simulink model "PubIfDecisionTOS_MDL"  (R2020b)
settings: configuration reference "DspaceConfig" (kept outside this file)
PostLoadFcn:
  | if any(exist('dsrtsu_mdlpostloadfcn', 'file') ~= 0), dsrtsu_mdlpostloadfcn('Execute', bdroot); end
InitFcn:
  | , if any(exist('dsmpb_private', 'file') ~= 0), dsmpb_private('dsmpb_mdlclblib', 'Init', bdroot); end,
undefined symbols (not defined in the file or in its folder): C_TOS_ACCEgoRAxletoFbumplength_m, C_TOS_ACCTargetFront_Flag, C_TOS_AEBJAPedObjDxThre_Val, C_TOS_AEBJAPedObjDyThre_Val, C_TOS_AEBJATargetSize_Val, C_TOS_AEBJAVehObjDxThre_Val, C_TOS_AEBJAVehObjDyThre_Val, C_TOS_AEBJuncPedTargetSize_Val, C_TOS_AEBLatObjDxThre_Val, C_TOS_AEBLatPedDyThre_Val, C_TOS_AEBLatTargetSize_Val, C_TOS_AEBLongTargetInEgoFront_Flag, C_TOS_axAbsGround_Parameter, C_TOS_CameraConfirmedFlag, C_TOS_CNsubjWidth, C_TOS_CurrentLaneCoreMinWidth_Val, C_TOS_CutInProb_Val_Zero, C_TOS_CutOutProb_Val_Zero, C_TOS_D2R_Val, C_TOS_DefaultValueObjectToCenterLine_dy, C_TOS_EgoCarWidth_Val, C_TOS_EgoDxRefPoint_m, C_TOS_EgoRAxletoFbumplength_m, C_TOS_HalfWidthVehicle_Con, C_TOS_HWA_CurrentLaneFlag, C_TOS_HWA_LeftLaneFlag, C_TOS_HWA_MovingDir_Vaild, C_TOS_HWA_MovState_Vaild, C_TOS_HWA_RightLaneFlag, C_TOS_LaneLineCourseErrorFront, C_TOS_LaneLineCourseErrorRear, C_TOS_MotorbikeDefaultWidth_m, C_TOS_NumberOfEffectiveTargets, C_TOS_Obj_Age_Val, C_TOS_Objdx_Constraint_Val, C_TOS_ObjectDefaultWidth_m, C_TOS_ObjInCurrentLane_Val, C_TOS_ObjInCurrentLaneValid, C_TOS_ObjInLeftLaneValid, C_TOS_ObjInRightLaneValid, C_TOS_ObjNotInCurrentLane_Val, C_TOS_ObjNotREElementType, C_TOS_ObjPredictDis_dy_ConstantVal_Zeros, C_TOS_ObjToCenterLine_ConstantVal_Zeros, C_TOS_OFMObjIDInvilad_Val, C_TOS_PIL_LatDisCons_Val_zero, C_TOS_PIL_ObjectCutInFlag_b, C_TOS_PIL_ObjectCutOutFlag_b, C_TOS_PIL_ObjLaneProb_al_Val, C_TOS_PP_ObjFusType_FC_Confirm_b, C_TOS_PP_ObjFusType_FC_FR_Confirm_b, C_TOS_PP_ObjFusType_FR_Confirm_b, C_TOS_RE_80BoolDefault_Val, C_TOS_RE_80Single181Default_Val, C_TOS_RE_80Single255Default_Val, C_TOS_RE_80Uint8Default_Val, C_TOS_RE_D2R, C_TOS_RE_D_180_Val, C_TOS_RE_InvalidObjectID_Val, C_TOS_RE_InvalidTargetChainDir_Val ... (+142)
libraries: simulink x1650, TOS_LIB x361, canfdmsglib x14
(part 32 of 69)

== system PubIfDecisionTOS_MDL/TOS_20201112/TOS_2012080320/PIL_1029/BoundaryCalculat/ObjectToCenterLine_dyc/RightLane/RightCenterLine_dyc/ObjToCenterLine_dyc_RightLane/line01_dy ==
  Object_DX : Inport
  line01_C0 : Inport  Port=2
  line01_C1 : Inport  Port=3
  line01_C2 : Inport  Port=4
  line01_C3 : Inport  Port=5
  Add : Sum
  Add1 : Sum
  Add3 : Sum
  Constant1 : Constant  Value=3  OutDataTypeStr=single
  Math Function1 : Math  Operator=pow  SignedPower=on  SaturateOnIntegerOverflow=on
  Product : Product
  Product1 : Product
  Product2 : Product
  Square : Math  Operator=square  SignedPower=on  SaturateOnIntegerOverflow=on
  line01_dy : Outport
  wires:
  line01_C1/1 -> Product1/2
  line01_C3/1 -> Product2/2
  Add3/1 -> line01_dy/1
  Add/1 -> Add3/1
  Constant1/1 -> Math Function1/2
  Product1/1 -> Add1/2
  Product2/1 -> Add3/2
  Math Function1/1 -> Product2/1
  Object_DX/1 -> Math Function1/1, Square/1, Product1/1
  Square/1 -> Product/1
  line01_C2/1 -> Product/2
  Product/1 -> Add/2
  line01_C0/1 -> Add1/1
  Add1/1 -> Add/1

== system PubIfDecisionTOS_MDL/TOS_20201112/TOS_2012080320/PIL_1029/BoundaryCalculat/ObjectToCenterLine_dyc/RightLane/RightCenterLine_dyc/ObjToCenterLine_dyc_RightLane/line02_DisJudge ==
  Object_DX : Inport
  line02_dDisStart : Inport  Port=2
  line02_dDisEnd : Inport  Port=3
  Logical Operator : Logic  AllPortsSameDT=off  OutDataTypeStr=boolean
  Relational Operator : RelationalOperator  OutDataTypeStr=boolean  RndMeth=Nearest
  Relational Operator1 : RelationalOperator  Operator=<  OutDataTypeStr=boolean  RndMeth=Nearest
  line02_DisJudge : Outport
  wires:
  Logical Operator/1 -> line02_DisJudge/1
  Relational Operator1/1 -> Logical Operator/2
  Relational Operator/1 -> Logical Operator/1
  Object_DX/1 -> Relational Operator/1, Relational Operator1/1
  line02_dDisStart/1 -> Relational Operator/2
  line02_dDisEnd/1 -> Relational Operator1/2

== system PubIfDecisionTOS_MDL/TOS_20201112/TOS_2012080320/PIL_1029/BoundaryCalculat/ObjectToCenterLine_dyc/RightLane/RightCenterLine_dyc/ObjToCenterLine_dyc_RightLane/line02_dy ==
  Object_DX : Inport
  line02_C0 : Inport  Port=2
  line02_C1 : Inport  Port=3
  line02_C2 : Inport  Port=4
  line02_C3 : Inport  Port=5
  Add : Sum
  Add1 : Sum
  Add3 : Sum
  Constant1 : Constant  Value=3  OutDataTypeStr=single
  Math Function1 : Math  Operator=pow  SignedPower=on  SaturateOnIntegerOverflow=on
  Product : Product
  Product1 : Product
  Product2 : Product
  Square : Math  Operator=square  SignedPower=on  SaturateOnIntegerOverflow=on
  line02_dy : Outport
  wires:
  Add1/1 -> Add/1
  line02_C0/1 -> Add1/1
  Product/1 -> Add/2
  line02_C2/1 -> Product/2
  Square/1 -> Product/1
  Object_DX/1 -> Product1/1, Square/1, Math Function1/1
  Math Function1/1 -> Product2/1
  Product2/1 -> Add3/2
  Product1/1 -> Add1/2
  Constant1/1 -> Math Function1/2
  Add/1 -> Add3/1
  Add3/1 -> line02_dy/1
  line02_C3/1 -> Product2/2
  line02_C1/1 -> Product1/2

== system PubIfDecisionTOS_MDL/TOS_20201112/TOS_2012080320/PIL_1029/BoundaryCalculat/ObjectToCenterLine_dyc/RightLane/RightCenterLine_dyc/ObjToCenterLine_dyc_RightLane/line03_DisJudge ==
  Object_DX : Inport
  line03_dDisStart : Inport  Port=2
  line03_dDisEnd : Inport  Port=3
  Logical Operator : Logic  AllPortsSameDT=off  OutDataTypeStr=boolean
  Relational Operator : RelationalOperator  OutDataTypeStr=boolean  RndMeth=Nearest
  Relational Operator1 : RelationalOperator  Operator=<  OutDataTypeStr=boolean  RndMeth=Nearest
  line03_DisJudge : Outport
  wires:
  line03_dDisEnd/1 -> Relational Operator1/2
  line03_dDisStart/1 -> Relational Operator/2
  Object_DX/1 -> Relational Operator1/1, Relational Operator/1
  Relational Operator/1 -> Logical Operator/1
  Relational Operator1/1 -> Logical Operator/2
  Logical Operator/1 -> line03_DisJudge/1

== system PubIfDecisionTOS_MDL/TOS_20201112/TOS_2012080320/PIL_1029/BoundaryCalculat/ObjectToCenterLine_dyc/RightLane/RightCenterLine_dyc/ObjToCenterLine_dyc_RightLane/line03_dy ==
  Object_DX : Inport
  line03_C0 : Inport  Port=2
  line03_C1 : Inport  Port=3
  line03_C2 : Inport  Port=4
  line03_C3 : Inport  Port=5
  Add : Sum
  Add1 : Sum
  Add3 : Sum
  Constant1 : Constant  Value=3  OutDataTypeStr=single
  Math Function1 : Math  Operator=pow  SignedPower=on  SaturateOnIntegerOverflow=on
  Product : Product
  Product1 : Product
  Product2 : Product
  Square : Math  Operator=square  SignedPower=on  SaturateOnIntegerOverflow=on
  line03_dy : Outport
  wires:
  line03_C1/1 -> Product1/2
  line03_C3/1 -> Product2/2
  Add3/1 -> line03_dy/1
  Add/1 -> Add3/1
  Constant1/1 -> Math Function1/2
  Product1/1 -> Add1/2
  Product2/1 -> Add3/2
  Math Function1/1 -> Product2/1
  Object_DX/1 -> Math Function1/1, Square/1, Product1/1
  Square/1 -> Product/1
  line03_C2/1 -> Product/2
  Product/1 -> Add/2
  line03_C0/1 -> Add1/1
  Add1/1 -> Add/1

== system PubIfDecisionTOS_MDL/TOS_20201112/TOS_2012080320/PIL_1029/BoundaryCalculat/ObjectToCenterLine_dyc/RightLane/RightCenterLine_dyc/ObjToCenterLine_dyc_RightLane/line04_DisJudge ==
  Object_DX : Inport
  line04_dDisStart : Inport  Port=2
  line04_dDisEnd : Inport  Port=3
  Logical Operator : Logic  AllPortsSameDT=off  OutDataTypeStr=boolean
  Relational Operator : RelationalOperator  OutDataTypeStr=boolean  RndMeth=Nearest
  Relational Operator1 : RelationalOperator  Operator=<  OutDataTypeStr=boolean  RndMeth=Nearest
  line04_DisJudge : Outport
  wires:
  Logical Operator/1 -> line04_DisJudge/1
  Relational Operator1/1 -> Logical Operator/2
  Relational Operator/1 -> Logical Operator/1
  Object_DX/1 -> Relational Operator/1, Relational Operator1/1
  line04_dDisStart/1 -> Relational Operator/2
  line04_dDisEnd/1 -> Relational Operator1/2

== system PubIfDecisionTOS_MDL/TOS_20201112/TOS_2012080320/PIL_1029/BoundaryCalculat/ObjectToCenterLine_dyc/RightLane/RightCenterLine_dyc/ObjToCenterLine_dyc_RightLane/line04_dy ==
  Object_DX : Inport
  line04_C0 : Inport  Port=2
  line04_C1 : Inport  Port=3
  line04_C2 : Inport  Port=4
  line04_C3 : Inport  Port=5
  Add : Sum
  Add1 : Sum
  Add3 : Sum
  Constant1 : Constant  Value=3  OutDataTypeStr=single
  Math Function1 : Math  Operator=pow  SignedPower=on  SaturateOnIntegerOverflow=on
  Product : Product
  Product1 : Product
  Product2 : Product
  Square : Math  Operator=square  SignedPower=on  SaturateOnIntegerOverflow=on
  line04_dy : Outport
  wires:
  Add1/1 -> Add/1
  line04_C0/1 -> Add1/1
  Product/1 -> Add/2
  line04_C2/1 -> Product/2
  Square/1 -> Product/1
  Object_DX/1 -> Product1/1, Square/1, Math Function1/1
  Math Function1/1 -> Product2/1
  Product2/1 -> Add3/2
  Product1/1 -> Add1/2
  Constant1/1 -> Math Function1/2
  Add/1 -> Add3/1
  Add3/1 -> line04_dy/1
  line04_C3/1 -> Product2/2
  line04_C1/1 -> Product1/2

== system PubIfDecisionTOS_MDL/TOS_20201112/TOS_2012080320/PIL_1029/BoundaryCalculat/ObjectToCenterLine_dyc/RightLane/RightCenterLine_dyc/ObjToCenterLine_dyc_RightLane/line05_DisJudge ==
  Object_DX : Inport
  line05_dDisStart : Inport  Port=2
  line05_dDisEnd : Inport  Port=3
  Logical Operator : Logic  AllPortsSameDT=off  OutDataTypeStr=boolean
  Relational Operator : RelationalOperator  OutDataTypeStr=boolean  RndMeth=Nearest
  Relational Operator1 : RelationalOperator  Operator=<  OutDataTypeStr=boolean  RndMeth=Nearest
  line05_DisJudge : Outport
  wires:
  line05_dDisEnd/1 -> Relational Operator1/2
  line05_dDisStart/1 -> Relational Operator/2
  Object_DX/1 -> Relational Operator1/1, Relational Operator/1
  Relational Operator/1 -> Logical Operator/1
  Relational Operator1/1 -> Logical Operator/2
  Logical Operator/1 -> line05_DisJudge/1

== system PubIfDecisionTOS_MDL/TOS_20201112/TOS_2012080320/PIL_1029/BoundaryCalculat/ObjectToCenterLine_dyc/RightLane/RightCenterLine_dyc/ObjToCenterLine_dyc_RightLane/line05_dy ==
  Object_DX : Inport
  line05_C0 : Inport  Port=2
  line05_C1 : Inport  Port=3
  line05_C2 : Inport  Port=4
  line05_C3 : Inport  Port=5
  Add : Sum
  Add1 : Sum
  Add3 : Sum
  Constant1 : Constant  Value=3  OutDataTypeStr=single
  Math Function1 : Math  Operator=pow  SignedPower=on  SaturateOnIntegerOverflow=on
  Product : Product
  Product1 : Product
  Product2 : Product
  Square : Math  Operator=square  SignedPower=on  SaturateOnIntegerOverflow=on
  line05_dy : Outport
  wires:
  line05_C1/1 -> Product1/2
  line05_C3/1 -> Product2/2
  Add3/1 -> line05_dy/1
  Add/1 -> Add3/1
  Constant1/1 -> Math Function1/2
  Product1/1 -> Add1/2
  Product2/1 -> Add3/2
  Math Function1/1 -> Product2/1
  Object_DX/1 -> Math Function1/1, Square/1, Product1/1
  Square/1 -> Product/1
  line05_C2/1 -> Product/2
  Product/1 -> Add/2
  line05_C0/1 -> Add1/1
  Add1/1 -> Add/1

== system PubIfDecisionTOS_MDL/TOS_20201112/TOS_2012080320/PIL_1029/BoundaryCalculat/ObjectToCenterLine_dyc/RightLane/RightCenterLine_dyc/ObjToCenterLine_dyc_RightLane/line06_DisJudge ==
  Object_DX : Inport
  line06_dDisStart : Inport  Port=2
  line06_dDisEnd : Inport  Port=3
  Logical Operator : Logic  AllPortsSameDT=off  OutDataTypeStr=boolean
  Relational Operator : RelationalOperator  OutDataTypeStr=boolean  RndMeth=Nearest
  Relational Operator1 : RelationalOperator  Operator=<  OutDataTypeStr=boolean  RndMeth=Nearest
  line06_DisJudge : Outport
  wires:
  Logical Operator/1 -> line06_DisJudge/1
  Relational Operator1/1 -> Logical Operator/2
  Relational Operator/1 -> Logical Operator/1
  Object_DX/1 -> Relational Operator/1, Relational Operator1/1
  line06_dDisStart/1 -> Relational Operator/2
  line06_dDisEnd/1 -> Relational Operator1/2

== system PubIfDecisionTOS_MDL/TOS_20201112/TOS_2012080320/PIL_1029/BoundaryCalculat/ObjectToCenterLine_dyc/RightLane/RightCenterLine_dyc/ObjToCenterLine_dyc_RightLane/line06_dy ==
  Object_DX : Inport
  line06_C0 : Inport  Port=2
  line06_C1 : Inport  Port=3
  line06_C2 : Inport  Port=4
  line6_C3 : Inport  Port=5
  Add : Sum
  Add1 : Sum
  Add3 : Sum
  Constant1 : Constant  Value=3  OutDataTypeStr=single
  Math Function1 : Math  Operator=pow  SignedPower=on  SaturateOnIntegerOverflow=on
  Product : Product
  Product1 : Product
  Product2 : Product
  Square : Math  Operator=square  SignedPower=on  SaturateOnIntegerOverflow=on
  line6_dy : Outport
  wires:
  Add1/1 -> Add/1
  line06_C0/1 -> Add1/1
  Product/1 -> Add/2
  line06_C2/1 -> Product/2
  Square/1 -> Product/1
  Object_DX/1 -> Product1/1, Square/1, Math Function1/1
  Math Function1/1 -> Product2/1
  Product2/1 -> Add3/2
  Product1/1 -> Add1/2
  Constant1/1 -> Math Function1/2
  Add/1 -> Add3/1
  Add3/1 -> line6_dy/1
  line6_C3/1 -> Product2/2
  line06_C1/1 -> Product1/2

== system PubIfDecisionTOS_MDL/TOS_20201112/TOS_2012080320/PIL_1029/BoundaryCalculat/ObjectToCenterLine_dyc/SameLane/PIL_ObjectToCenterLine_dy_Filt/PIL_ObjectToCenterLine_dy/PP_SignalProcessingDefault ==
  Action Port : ActionPort  ActionPortLabel=if(u1 ~= 0)
  Constant : Constant  Value=0  OutDataTypeStr=uint8
  Constant1 : Constant  Value=255  OutDataTypeStr=single
  Obj_ID : Outport
  ObjectToCenterLine_dy_Filt : Outport  Port=2  OutDataTypeStr=single
  wires:
  Constant1/1 -> ObjectToCenterLine_dy_Filt/1
  Constant/1 -> Obj_ID/1

== system PubIfDecisionTOS_MDL/TOS_20201112/TOS_2012080320/PIL_1029/BoundaryCalculat/ObjectToCenterLine_dyc/SameLane/PIL_ObjectToCenterLine_dy_Filt/PIL_ObjectToCenterLine_dy/Subsystem ==
  ObjectID_Filt_K1 : Inport
  ObjectToCenterLine_dy_Filt_K1 : Inport  Port=2  OutDataTypeStr=single
  ObjectToCenterLine_dy : Inport  Port=3  OutDataTypeStr=single
  Object_ID : Inport  Port=4  OutDataTypeStr=uint8
  Object_Age : Inport  Port=5
  TOS_OFMObjValid_Flag : Inport  Port=6
  Action Port : ActionPort  ActionPortLabel=else
  Constant1 : Constant  Value=C_TOS_NumberOfEffectiveTargets  OutDataTypeStr=int32
      settings: AttributesFormatString=C_TOS_NumberOfEffectiveTargets = 80
  Constant2 : Constant  Value=0.2  OutDataTypeStr=single
      settings: AttributesFormatString=P_TOS_PIL_ObjectToCenterLine_dy_CutInDeclineLimit = 0.1
  Constant8 : Constant  Value=0.35  OutDataTypeStr=single
      settings: AttributesFormatString=P_TOS_PIL_ObjectToCenterLine_dy_CutInUpperLimit = 0.5
  ObjectToCenterLine_dyFilit : MATLAB Function  TreatAsAtomicUnit=on
  Terminator : Terminator
  Obj_ID : Outport
  ObjectToCenterLine_dy_Filt : Outport  Port=2  OutDataTypeStr=single
  wires:
  TOS_OFMObjValid_Flag/1 -> ObjectToCenterLine_dyFilit/5(TOS_OFMObjValid_Flag)
  Object_Age/1 -> Terminator/1
  ObjectToCenterLine_dy_Filt_K1/1 -> ObjectToCenterLine_dyFilit/2(ObjectToCenterLine_dy_Filt_K1)
  Object_ID/1 -> Obj_ID/1, ObjectToCenterLine_dyFilit/4(Object_ID)
  ObjectID_Filt_K1/1 -> ObjectToCenterLine_dyFilit/1(ObjectID_Filt_K1)
  Constant2/1 -> ObjectToCenterLine_dyFilit/7(P_TOS_PIL_ObjectToCenterLine_dy_CutInDeclineLimit)
  Constant1/1 -> ObjectToCenterLine_dyFilit/8(Iterator_Num)
  ObjectToCenterLine_dy/1 -> ObjectToCenterLine_dyFilit/3(ObjectToCenterLine_dy)
  Constant8/1 -> ObjectToCenterLine_dyFilit/6(P_TOS_PIL_ObjectToCenterLine_dy_CutInUpperLimit)
  ObjectToCenterLine_dyFilit/1(ObjectToCenterLine_dy_Filt) -> ObjectToCenterLine_dy_Filt/1

== system PubIfDecisionTOS_MDL/TOS_20201112/TOS_2012080320/PIL_1029/BoundaryCalculat/ObjectToCenterLine_dyc/SameLane/SameCenterLine_dyc/ObjToCenterLine_dyc_CurrentLane/line01_DisJudge ==
  Object_DX : Inport
  line01_dDisStart : Inport  Port=2
  line01_dDisEnd : Inport  Port=3
  Logical Operator : Logic  AllPortsSameDT=off  OutDataTypeStr=boolean
  Relational Operator : RelationalOperator  OutDataTypeStr=boolean  RndMeth=Nearest
  Relational Operator1 : RelationalOperator  Operator=<  OutDataTypeStr=boolean  RndMeth=Nearest
  line01_DisJudge : Outport
  wires:
  Logical Operator/1 -> line01_DisJudge/1
  Relational Operator1/1 -> Logical Operator/2
  Relational Operator/1 -> Logical Operator/1
  Object_DX/1 -> Relational Operator/1, Relational Operator1/1
  line01_dDisStart/1 -> Relational Operator/2
  line01_dDisEnd/1 -> Relational Operator1/2

== system PubIfDecisionTOS_MDL/TOS_20201112/TOS_2012080320/PIL_1029/BoundaryCalculat/ObjectToCenterLine_dyc/SameLane/SameCenterLine_dyc/ObjToCenterLine_dyc_CurrentLane/line01_dy ==
  Object_DX : Inport
  line01_C0 : Inport  Port=2
  line01_C1 : Inport  Port=3
  line01_C2 : Inport  Port=4
  line01_C3 : Inport  Port=5
  Add : Sum
  Add1 : Sum
  Add3 : Sum
  Constant1 : Constant  Value=3  OutDataTypeStr=single
  Math Function1 : Math  Operator=pow  SignedPower=on  SaturateOnIntegerOverflow=on
  Product : Product
  Product1 : Product
  Product2 : Product
  Square : Math  Operator=square  SignedPower=on  SaturateOnIntegerOverflow=on
  line01_dy : Outport
  wires:
  Add1/1 -> Add/1
  line01_C0/1 -> Add1/1
  Product/1 -> Add/2
  line01_C2/1 -> Product/2
  Square/1 -> Product/1
  Object_DX/1 -> Product1/1, Square/1, Math Function1/1
  Math Function1/1 -> Product2/1
  Product2/1 -> Add3/2
  Product1/1 -> Add1/2
  Constant1/1 -> Math Function1/2
  Add/1 -> Add3/1
  Add3/1 -> line01_dy/1
  line01_C3/1 -> Product2/2
  line01_C1/1 -> Product1/2

== system PubIfDecisionTOS_MDL/TOS_20201112/TOS_2012080320/PIL_1029/BoundaryCalculat/ObjectToCenterLine_dyc/SameLane/SameCenterLine_dyc/ObjToCenterLine_dyc_CurrentLane/line02_DisJudge ==
  Object_DX : Inport
  line02_dDisStart : Inport  Port=2
  line02_dDisEnd : Inport  Port=3
  Logical Operator : Logic  AllPortsSameDT=off  OutDataTypeStr=boolean
  Relational Operator : RelationalOperator  OutDataTypeStr=boolean  RndMeth=Nearest
  Relational Operator1 : RelationalOperator  Operator=<  OutDataTypeStr=boolean  RndMeth=Nearest
  line02_DisJudge : Outport
  wires:
  line02_dDisEnd/1 -> Relational Operator1/2
  line02_dDisStart/1 -> Relational Operator/2
  Object_DX/1 -> Relational Operator1/1, Relational Operator/1
  Relational Operator/1 -> Logical Operator/1
  Relational Operator1/1 -> Logical Operator/2
  Logical Operator/1 -> line02_DisJudge/1

== system PubIfDecisionTOS_MDL/TOS_20201112/TOS_2012080320/PIL_1029/BoundaryCalculat/ObjectToCenterLine_dyc/SameLane/SameCenterLine_dyc/ObjToCenterLine_dyc_CurrentLane/line02_dy ==
  Object_DX : Inport
  line02_C0 : Inport  Port=2
  line02_C1 : Inport  Port=3
  line02_C2 : Inport  Port=4
  line02_C3 : Inport  Port=5
  Add : Sum
  Add1 : Sum
  Add3 : Sum
  Constant1 : Constant  Value=3  OutDataTypeStr=single
  Math Function1 : Math  Operator=pow  SignedPower=on  SaturateOnIntegerOverflow=on
  Product : Product
  Product1 : Product
  Product2 : Product
  Square : Math  Operator=square  SignedPower=on  SaturateOnIntegerOverflow=on
  line02_dy : Outport
  wires:
  line02_C1/1 -> Product1/2
  line02_C3/1 -> Product2/2
  Add3/1 -> line02_dy/1
  Add/1 -> Add3/1
  Constant1/1 -> Math Function1/2
  Product1/1 -> Add1/2
  Product2/1 -> Add3/2
  Math Function1/1 -> Product2/1
  Object_DX/1 -> Math Function1/1, Square/1, Product1/1
  Square/1 -> Product/1
  line02_C2/1 -> Product/2
  Product/1 -> Add/2
  line02_C0/1 -> Add1/1
  Add1/1 -> Add/1

== system PubIfDecisionTOS_MDL/TOS_20201112/TOS_2012080320/PIL_1029/BoundaryCalculat/ObjectToCenterLine_dyc/SameLane/SameCenterLine_dyc/ObjToCenterLine_dyc_CurrentLane/line03_DisJudge ==
  Object_DX : Inport
  line03_dDisStart : Inport  Port=2
  line03_dDisEnd : Inport  Port=3
  Logical Operator : Logic  AllPortsSameDT=off  OutDataTypeStr=boolean
  Relational Operator : RelationalOperator  OutDataTypeStr=boolean  RndMeth=Nearest
  Relational Operator1 : RelationalOperator  Operator=<  OutDataTypeStr=boolean  RndMeth=Nearest
  line03_DisJudge : Outport
  wires:
  Logical Operator/1 -> line03_DisJudge/1
  Relational Operator1/1 -> Logical Operator/2
  Relational Operator/1 -> Logical Operator/1
  Object_DX/1 -> Relational Operator/1, Relational Operator1/1
  line03_dDisStart/1 -> Relational Operator/2
  line03_dDisEnd/1 -> Relational Operator1/2

== system PubIfDecisionTOS_MDL/TOS_20201112/TOS_2012080320/PIL_1029/BoundaryCalculat/ObjectToCenterLine_dyc/SameLane/SameCenterLine_dyc/ObjToCenterLine_dyc_CurrentLane/line03_dy ==
  Object_DX : Inport
  line03_C0 : Inport  Port=2
  line03_C1 : Inport  Port=3
  line03_C2 : Inport  Port=4
  line03_C3 : Inport  Port=5
  Add : Sum
  Add1 : Sum
  Add3 : Sum
  Constant1 : Constant  Value=3  OutDataTypeStr=single
  Math Function1 : Math  Operator=pow  SignedPower=on  SaturateOnIntegerOverflow=on
  Product : Product
  Product1 : Product
  Product2 : Product
  Square : Math  Operator=square  SignedPower=on  SaturateOnIntegerOverflow=on
  line03_dy : Outport
  wires:
  Add1/1 -> Add/1
  line03_C0/1 -> Add1/1
  Product/1 -> Add/2
  line03_C2/1 -> Product/2
  Square/1 -> Product/1
  Object_DX/1 -> Product1/1, Square/1, Math Function1/1
  Math Function1/1 -> Product2/1
  Product2/1 -> Add3/2
  Product1/1 -> Add1/2
  Constant1/1 -> Math Function1/2
  Add/1 -> Add3/1
  Add3/1 -> line03_dy/1
  line03_C3/1 -> Product2/2
  line03_C1/1 -> Product1/2

== system PubIfDecisionTOS_MDL/TOS_20201112/TOS_2012080320/PIL_1029/BoundaryCalculat/ObjectToCenterLine_dyc/SameLane/SameCenterLine_dyc/ObjToCenterLine_dyc_CurrentLane/line04_DisJudge ==
  Object_DX : Inport
  line04_dDisStart : Inport  Port=2
  line04_dDisEnd : Inport  Port=3
  Logical Operator : Logic  AllPortsSameDT=off  OutDataTypeStr=boolean
  Relational Operator : RelationalOperator  OutDataTypeStr=boolean  RndMeth=Nearest
  Relational Operator1 : RelationalOperator  Operator=<  OutDataTypeStr=boolean  RndMeth=Nearest
  line04_DisJudge : Outport
  wires:
  line04_dDisEnd/1 -> Relational Operator1/2
  line04_dDisStart/1 -> Relational Operator/2
  Object_DX/1 -> Relational Operator1/1, Relational Operator/1
  Relational Operator/1 -> Logical Operator/1
  Relational Operator1/1 -> Logical Operator/2
  Logical Operator/1 -> line04_DisJudge/1

== system PubIfDecisionTOS_MDL/TOS_20201112/TOS_2012080320/PIL_1029/BoundaryCalculat/ObjectToCenterLine_dyc/SameLane/SameCenterLine_dyc/ObjToCenterLine_dyc_CurrentLane/line04_dy ==
  Object_DX : Inport
  line04_C0 : Inport  Port=2
  line04_C1 : Inport  Port=3
  line04_C2 : Inport  Port=4
  line04_C3 : Inport  Port=5
  Add : Sum
  Add1 : Sum
  Add3 : Sum
  Constant1 : Constant  Value=3  OutDataTypeStr=single
  Math Function1 : Math  Operator=pow  SignedPower=on  SaturateOnIntegerOverflow=on
  Product : Product
  Product1 : Product
  Product2 : Product
  Square : Math  Operator=square  SignedPower=on  SaturateOnIntegerOverflow=on
  line04_dy : Outport
  wires:
  line04_C1/1 -> Product1/2
  line04_C3/1 -> Product2/2
  Add3/1 -> line04_dy/1
  Add/1 -> Add3/1
  Constant1/1 -> Math Function1/2
  Product1/1 -> Add1/2
  Product2/1 -> Add3/2
  Math Function1/1 -> Product2/1
  Object_DX/1 -> Math Function1/1, Square/1, Product1/1
  Square/1 -> Product/1
  line04_C2/1 -> Product/2
  Product/1 -> Add/2
  line04_C0/1 -> Add1/1
  Add1/1 -> Add/1

== system PubIfDecisionTOS_MDL/TOS_20201112/TOS_2012080320/PIL_1029/BoundaryCalculat/ObjectToCenterLine_dyc/SameLane/SameCenterLine_dyc/ObjToCenterLine_dyc_CurrentLane/line05_DisJudge ==
  Object_DX : Inport
  line05_dDisStart : Inport  Port=2
  line05_dDisEnd : Inport  Port=3
  Logical Operator : Logic  AllPortsSameDT=off  OutDataTypeStr=boolean
  Relational Operator : RelationalOperator  OutDataTypeStr=boolean  RndMeth=Nearest
  Relational Operator1 : RelationalOperator  Operator=<  OutDataTypeStr=boolean  RndMeth=Nearest
  line05_DisJudge : Outport
  wires:
  Logical Operator/1 -> line05_DisJudge/1
  Relational Operator1/1 -> Logical Operator/2
  Relational Operator/1 -> Logical Operator/1
  Object_DX/1 -> Relational Operator/1, Relational Operator1/1
  line05_dDisStart/1 -> Relational Operator/2
  line05_dDisEnd/1 -> Relational Operator1/2

== system PubIfDecisionTOS_MDL/TOS_20201112/TOS_2012080320/PIL_1029/BoundaryCalculat/ObjectToCenterLine_dyc/SameLane/SameCenterLine_dyc/ObjToCenterLine_dyc_CurrentLane/line05_dy ==
  Object_DX : Inport
  line05_C0 : Inport  Port=2
  line05_C1 : Inport  Port=3
  line05_C2 : Inport  Port=4
  line05_C3 : Inport  Port=5
  Add : Sum
  Add1 : Sum
  Add3 : Sum
  Constant1 : Constant  Value=3  OutDataTypeStr=single
  Math Function1 : Math  Operator=pow  SignedPower=on  SaturateOnIntegerOverflow=on
  Product : Product
  Product1 : Product
  Product2 : Product
  Square : Math  Operator=square  SignedPower=on  SaturateOnIntegerOverflow=on
  line05_dy : Outport
  wires:
  Add1/1 -> Add/1
  line05_C0/1 -> Add1/1
  Product/1 -> Add/2
  line05_C2/1 -> Product/2
  Square/1 -> Product/1
  Object_DX/1 -> Product1/1, Square/1, Math Function1/1
  Math Function1/1 -> Product2/1
  Product2/1 -> Add3/2
  Product1/1 -> Add1/2
  Constant1/1 -> Math Function1/2
  Add/1 -> Add3/1
  Add3/1 -> line05_dy/1
  line05_C3/1 -> Product2/2
  line05_C1/1 -> Product1/2

== system PubIfDecisionTOS_MDL/TOS_20201112/TOS_2012080320/PIL_1029/BoundaryCalculat/ObjectToCenterLine_dyc/SameLane/SameCenterLine_dyc/ObjToCenterLine_dyc_CurrentLane/line06_DisJudge ==
  Object_DX : Inport
  line06_dDisStart : Inport  Port=2
  line06_dDisEnd : Inport  Port=3
  Logical Operator : Logic  AllPortsSameDT=off  OutDataTypeStr=boolean
  Relational Operator : RelationalOperator  OutDataTypeStr=boolean  RndMeth=Nearest
  Relational Operator1 : RelationalOperator  Operator=<  OutDataTypeStr=boolean  RndMeth=Nearest
  line06_DisJudge : Outport
  wires:
  line06_dDisEnd/1 -> Relational Operator1/2
  line06_dDisStart/1 -> Relational Operator/2
  Object_DX/1 -> Relational Operator1/1, Relational Operator/1
  Relational Operator/1 -> Logical Operator/1
  Relational Operator1/1 -> Logical Operator/2
  Logical Operator/1 -> line06_DisJudge/1

== system PubIfDecisionTOS_MDL/TOS_20201112/TOS_2012080320/PIL_1029/BoundaryCalculat/ObjectToCenterLine_dyc/SameLane/SameCenterLine_dyc/ObjToCenterLine_dyc_CurrentLane/line06_dy ==
  Object_DX : Inport
  line06_C0 : Inport  Port=2
  line06_C1 : Inport  Port=3
  line06_C2 : Inport  Port=4
  line6_C3 : Inport  Port=5
  Add : Sum
  Add1 : Sum
  Add3 : Sum
  Constant1 : Constant  Value=3  OutDataTypeStr=single
  Math Function1 : Math  Operator=pow  SignedPower=on  SaturateOnIntegerOverflow=on
  Product : Product
  Product1 : Product
  Product2 : Product
  Square : Math  Operator=square  SignedPower=on  SaturateOnIntegerOverflow=on
  line6_dy : Outport
  wires:
  line06_C1/1 -> Product1/2
  line6_C3/1 -> Product2/2
  Add3/1 -> line6_dy/1
  Add/1 -> Add3/1
  Constant1/1 -> Math Function1/2
  Product1/1 -> Add1/2
  Product2/1 -> Add3/2
  Math Function1/1 -> Product2/1
  Object_DX/1 -> Math Function1/1, Square/1, Product1/1
  Square/1 -> Product/1
  line06_C2/1 -> Product/2
  Product/1 -> Add/2
  line06_C0/1 -> Add1/1
  Add1/1 -> Add/1

== system PubIfDecisionTOS_MDL/TOS_20201112/TOS_2012080320/PIL_1029/ObjCutInOut_Prob/ObjectCutIn/CutInProb_Calculate/CutInProb_Calculate_/CutInPredictDis_dy/CutInPredictTime ==
  note: 非车辆目标，根据 ObjectToCenterLine_dy 定义预测时间
  ObjectToCenterLine_dy_Filt : Inport  OutDataTypeStr=single
  ObjectToCenterLine_dy : Inport  Port=2  OutDataTypeStr=single
  ObjectType : Inport  Port=3
  PP_ObjectToCenterLine_vyc : Inport  Port=4  OutDataTypeStr=single
  Object_DX : Inport  Port=5
  1-D Lookup Table : Lookup_n-D  NumberOfTableDimensions=1  BreakpointsForDimension1=[0,10,30,100]  Table=[1.35,1.35,1.35,1.35]  TableDataTypeStr=single  InternalRulePriority=Speed  RndMeth=Simplest  InputSameDT=on
  CarTruck_ToCenterLine_dy_Predict : Subsystem
  K_CutInMaxPredictTime_Val : Constant  Value=P_TOS_CutInMaxPredictTime_Val  OutDataTypeStr=single
      settings: AttributesFormatString=P_TOS_CutInMaxPredictTime_Val = 1.35
  K_CutInMinPredictTime_Val : Constant  Value=P_TOS_CutInMinPredictTime_Val  OutDataTypeStr=single
      settings: AttributesFormatString=P_TOS_CutInMinPredictTime_Val = 1.35
  ObjectToCenterLine_dy_Predict : Subsystem
  Switch : Switch  Criteria=u2 > Threshold  OutDataTypeStr=single
  Switch1 : Switch  Criteria=u2 > Threshold  OutDataTypeStr=single
  CutInPredictTime : Outport
  wires:
  K_CutInMaxPredictTime_Val/1 -> Switch/1
  K_CutInMinPredictTime_Val/1 -> Switch/3
  Switch/1 -> Switch1/3
  ObjectToCenterLine_dy_Filt/1 -> ObjectToCenterLine_dy_Predict/1(ObjectToCenterLine_dy_Filt)
  ObjectToCenterLine_dy/1 -> ObjectToCenterLine_dy_Predict/2(ObjectToCenterLine_dy)
  ObjectToCenterLine_dy_Predict/1(Out1) -> Switch/2
  ObjectType/1 -> CarTruck_ToCenterLine_dy_Predict/1(ObjectType)
  PP_ObjectToCenterLine_vyc/1 -> CarTruck_ToCenterLine_dy_Predict/2(PP_ObjectToCenterLine_vyc)
  CarTruck_ToCenterLine_dy_Predict/1(CarTruck_ToCenterLine_dy_Predict) -> Switch1/2
  Switch1/1 -> CutInPredictTime/1  "CutInPredictTime"
  1-D Lookup Table/1 -> Switch1/1  "CutInPredictTime"
  Object_DX/1 -> 1-D Lookup Table/1

== system PubIfDecisionTOS_MDL/TOS_20201112/TOS_2012080320/PIL_1029/ObjCutInOut_Prob/ObjectCutIn/CutInProb_Calculate/CutInProb_Calculate_/CutInPredictDis_dy/CutInPredictTime_Constraint ==
  note: fun:cut in 预测时间约束
      |
      | 根据 dx 约束目标预测时间
  note: [  min ,  prt ]
      | [  max , 0   ]
  note: 插值计算，根据dx距离 约束预测时间
  note: dx 距离约束范围：[ 3.93 , 110 ]
  CutInPredictTime : Inport
  Object_DX : Inport  Port=2
  Add1 : Sum  Inputs=+-  OutDataTypeStr=single
  Add2 : Sum  Inputs=-+  AccumDataTypeStr=single  OutDataTypeStr=single
  Compare To Constant : simulink/Logic and Bit Operations/Compare To Constant  relop=<=  const=P_TOS_CutInMinPredictDis_Val  OutDataTypeStr=boolean
      settings: AttributesFormatString=P_TOS_CutInMinPredictDis_Val = 3.93 m
  Compare To Constant1 : simulink/Logic and Bit Operations/Compare To Constant  relop=>=  const=P_TOS_CutInMaxPredictDis_Val  OutDataTypeStr=boolean
      settings: AttributesFormatString=P_TOS_CutInMaxPredictDis_Val = 110 m
  Divide : Product  Inputs=*/  OutDataTypeStr=single
  Divide1 : Product  Inputs=**  OutDataTypeStr=single
  Divide2 : Product  Inputs=**  OutDataTypeStr=single
  Divide3 : Product  Inputs=*/  OutDataTypeStr=single
  K_CutInMaxPredictDis_Val : Constant  Value=P_TOS_CutInMaxPredictDis_Val  OutDataTypeStr=single
      settings: AttributesFormatString=P_TOS_CutInMaxPredictDis_Val = 110
  K_CutInMinPredictDis_Val : Constant  Value=P_TOS_CutInMinPredictDis_Val  OutDataTypeStr=single
      settings: AttributesFormatString=P_TOS_CutInMinPredictDis_Val = 3.93
  Switch1 : Switch  Criteria=u2 > Threshold
  Switch2 : Switch  Criteria=u2 > Threshold
  CutInPredictTime_Constraint : Outport  OutDataTypeStr=single
  wires:
  Add1/1 -> Divide3/2, Divide/2
  K_CutInMaxPredictDis_Val/1 -> Switch2/1, [K_CutInMaxPredictDis_Val]
  CutInPredictTime/1 -> Divide/1, Divide2/1
  [K_CutInMaxPredictDis_Val] -> Add1/2
  Object_DX/1 -> Compare To Constant/1, Compare To Constant1/1, Switch2/3
  Divide/1 -> Divide1/1
  Divide2/1 -> Divide3/1
  K_CutInMinPredictDis_Val/1 -> [K_CutInMinPredictDis_Val], Switch1/1
  Switch1/1 -> Divide1/2
  [K_CutInMinPredictDis_Val] -> Add1/1
  Switch2/1 -> Switch1/3
  Compare To Constant/1 -> Switch1/2
  Divide1/1 -> Add2/2
  [K_CutInMaxPredictDis_Val] -> Divide2/2
  Divide3/1 -> Add2/1
  Add2/1 -> CutInPredictTime_Constraint/1
  Compare To Constant1/1 -> Switch2/2

== system PubIfDecisionTOS_MDL/TOS_20201112/TOS_2012080320/PIL_1029/ObjCutInOut_Prob/ObjectCutIn/CutInProb_Calculate/CutInProb_Calculate_/CutInPredictDis_dy/CutInPredictTime_Constraint2 ==
  note: 目标由左→右；过线
  note: 预测距离dy'
  note: 当前距离dy + 预测距离dy'
  note: 目标由右→左；过线
  ObjectToCenterLine_dy : Inport
  CutInPredictTime_Constraint : Inport  Port=2
  PP_ObjectToCenterLine_vyc : Inport  Port=3
  Add3 : Sum  OutDataTypeStr=single
  Compare To Constant : simulink/Logic and Bit Operations/Compare To Constant  relop=<  const=C_TOS_ObjToCenterLine_ConstantVal_Zeros  OutDataTypeStr=boolean
      settings: AttributesFormatString=C_TOS_ObjToCenterLine_ConstantVal_Zeros = 0
  Compare To Constant1 : simulink/Logic and Bit Operations/Compare To Constant  relop=>  const=C_TOS_ObjToCenterLine_ConstantVal_Zeros  OutDataTypeStr=boolean
      settings: AttributesFormatString=C_TOS_ObjToCenterLine_ConstantVal_Zeros = 0
  Compare To Constant2 : simulink/Logic and Bit Operations/Compare To Constant  relop=>  const=C_TOS_ObjToCenterLine_ConstantVal_Zeros  OutDataTypeStr=boolean
      settings: AttributesFormatString=C_TOS_ObjToCenterLine_ConstantVal_Zeros = 0
  Compare To Constant3 : simulink/Logic and Bit Operations/Compare To Constant  relop=<  const=C_TOS_ObjToCenterLine_ConstantVal_Zeros  OutDataTypeStr=boolean
      settings: AttributesFormatString=C_TOS_ObjToCenterLine_ConstantVal_Zeros = 0
  Compare To Constant4 : simulink/Logic and Bit Operations/Compare To Constant  relop===  const=C_TOS_ObjToCenterLine_ConstantVal_Zeros  OutDataTypeStr=boolean
      settings: AttributesFormatString=C_TOS_ObjToCenterLine_ConstantVal_Zeros = 0
  Constant2 : Constant  Value=C_TOS_ObjPredictDis_dy_ConstantVal_Zeros  OutDataTypeStr=single
      settings: AttributesFormatString=C_TOS_ObjPredictDis_dy_ConstantVal_Zeros = 0
  Constant5 : Constant  Value=C_TOS_ObjPredictDis_dy_ConstantVal_Zeros  OutDataTypeStr=single
      settings: AttributesFormatString=C_TOS_ObjPredictDis_dy_ConstantVal_Zeros = 0
  Constant6 : Constant  Value=C_TOS_ObjPredictDis_dy_ConstantVal_Zeros  OutDataTypeStr=single
      settings: AttributesFormatString=C_TOS_ObjPredictDis_dy_ConstantVal_Zeros = 0
  Divide4 : Product  Inputs=**  OutDataTypeStr=single
  Logical Operator3 : Logic  AllPortsSameDT=off  OutDataTypeStr=boolean
  Logical Operator4 : Logic  AllPortsSameDT=off  OutDataTypeStr=boolean
  Switch3 : Switch  Criteria=u2 > Threshold  OutDataTypeStr=single
  Switch4 : Switch  Criteria=u2 > Threshold  OutDataTypeStr=single
  Switch5 : Switch  Criteria=u2 > Threshold  OutDataTypeStr=single
  CutInPredictDis_dy : Outport  OutDataTypeStr=single
  wires:
  Compare To Constant/1 -> Logical Operator3/1
  Logical Operator3/1 -> Switch3/2
  Constant5/1 -> Switch5/1
  PP_ObjectToCenterLine_vyc/1 -> Divide4/2
  Add3/1 -> Compare To Constant/1, Switch5/3, Compare To Constant2/1
  Logical Operator4/1 -> Switch4/2
  Divide4/1 -> Add3/1
  ObjectToCenterLine_dy/1 -> [ObjectToCenterLine_dy], Add3/2
  [ObjectToCenterLine_dy] -> Compare To Constant4/1
  Compare To Constant3/1 -> Logical Operator4/2
  [ObjectToCenterLine_dy] -> Compare To Constant3/1
  Switch3/1 -> CutInPredictDis_dy/1
  Compare To Constant4/1 -> Switch5/2
  Constant2/1 -> Switch3/1
  Switch5/1 -> Switch4/3
  Compare To Constant1/1 -> Logical Operator3/2
  Constant6/1 -> Switch4/1
  [ObjectToCenterLine_dy] -> Compare To Constant1/1
  Compare To Constant2/1 -> Logical Operator4/1
  Switch4/1 -> Switch3/3
  CutInPredictTime_Constraint/1 -> Divide4/1

== system PubIfDecisionTOS_MDL/TOS_20201112/TOS_2012080320/PIL_1029/ObjCutInOut_Prob/ObjectCutIn/CutInProb_Calculate/CutInProb_Calculate_/CutInProb/CutInObjWidthConstraint ==
  note: 根据目标宽度，修正切入预测距离
  note: 目标在中心线左侧
  note: 目标在中心线右侧
  CutInPredictDis_dy : Inport  OutDataTypeStr=single
  ObjectToCenterLine_dy : Inport  Port=2  OutDataTypeStr=single
  Object_Width : Inport  Port=3
  ObjectType : Inport  Port=4
  Add : Sum  Inputs=-+
  Add1 : Sum
  C_HalfWidthVehicle_Con : Constant  Value=C_TOS_HalfWidthVehicle_Con  OutDataTypeStr=single
      settings: AttributesFormatString=C_TOS_HalfWidthVehicle_Con = 0.5
  Constant3 : Constant  Value=C_TOS_ObjToCenterLine_ConstantVal_Zeros  OutDataTypeStr=single
      settings: AttributesFormatString=C_TOS_ObjToCenterLine_ConstantVal_Zeros = 0
  Max : MinMax  Function=max  Inputs=2  OutDataTypeStr=single
  Max1 : MinMax  Inputs=2  OutDataTypeStr=single
  ObjectWidth_Check : Subsystem
  Product : Product  OutDataTypeStr=single
  Relational Operator : RelationalOperator  Operator=>  OutDataTypeStr=boolean  RndMeth=Nearest
  Switch : Switch  Criteria=u2 > Threshold  OutDataTypeStr=single
  constant1 : Constant  Value=0  OutDataTypeStr=single
  constant2 : Constant  Value=0  OutDataTypeStr=single
  CutInPredictDis_dy_ObjWidthConstraint : Outport
  wires:
  ObjectType/1 -> ObjectWidth_Check/1(ObjectType)
  Object_Width/1 -> ObjectWidth_Check/2(Object_Width)
  Add1/1 -> Max1/2
  Product/1 -> Add/1, Add1/2
  C_HalfWidthVehicle_Con/1 -> Product/1
  Relational Operator/1 -> Switch/2
  ObjectToCenterLine_dy/1 -> Relational Operator/1
  Constant3/1 -> Relational Operator/2
  constant1/1 -> Max/1
  CutInPredictDis_dy/1 -> Add/2, Add1/1
  ObjectWidth_Check/1(ObjectWidth) -> Product/2
  Max/1 -> Switch/1
  constant2/1 -> Max1/1
  Max1/1 -> Switch/3
  Add/1 -> Max/2
  Switch/1 -> CutInPredictDis_dy_ObjWidthConstraint/1

== system PubIfDecisionTOS_MDL/TOS_20201112/TOS_2012080320/PIL_1029/ObjCutInOut_Prob/ObjectCutIn/CutInProb_Calculate/CutInProb_Calculate_/CutInProb/CutInProb_Calculation ==
  note: 当前值 + 预测值 ；
  note: 预测时机修正
  CutInPredictDis_dy_ObjWidthConstraint : Inport
  Abs : Abs
  Add2 : Sum  Inputs=+-  OutDataTypeStr=single
  Add4 : Sum  Inputs=+-  OutDataTypeStr=single
  Compare To Constant1 : simulink/Logic and Bit Operations/Compare To Constant  relop=>=  const=P_TOS_CutInMaxPredict_dy_Val  OutDataTypeStr=boolean
      settings: AttributesFormatString=P_TOS_CutInMaxPredict_dy_Val = 1.2
  Compare To Constant2 : simulink/Logic and Bit Operations/Compare To Constant  relop=<=  const=P_TOS_CutInMinPredict_dy_Val  OutDataTypeStr=boolean
      settings: AttributesFormatString=P_TOS_CutInMinPredict_dy_Val = 0
  Divide : Product  Inputs=*/  OutDataTypeStr=single
  Divide3 : Product  Inputs=*/  OutDataTypeStr=single
  K_CutInMaxPredict_dy_Val : Constant  Value=P_TOS_CutInMaxPredict_dy_Val  OutDataTypeStr=single
      settings: AttributesFormatString=P_TOS_CutInMaxPredict_dy_Val = 1.2
  K_CutInMinPredict_dy_Val : Constant  Value=P_TOS_CutInMinPredict_dy_Val  OutDataTypeStr=single
      settings: AttributesFormatString="P_TOS_CutInMinPredict_dy_Val  = 0"
  Switch1 : Switch  Criteria=u2 > Threshold
  Switch2 : Switch  Criteria=u2 > Threshold
  CutInProb_Calculation : Outport
  wires:
  CutInPredictDis_dy_ObjWidthConstraint/1 -> Abs/1
  Divide3/1 -> Add4/2
  Switch2/1 -> Switch1/3
  K_CutInMaxPredict_dy_Val/1 -> [K_CutInMaxPredict_dy_Val], Switch2/1
  Switch1/1 -> Divide/1
  Divide/1 -> Add4/1
  [K_CutInMaxPredict_dy_Val] -> Divide3/1
  [K_CutInMinPredict_dy_Val] -> Add2/1
  [K_CutInMaxPredict_dy_Val] -> Add2/2
  Add2/1 -> Divide3/2, Divide/2
  K_CutInMinPredict_dy_Val/1 -> Switch1/1, [K_CutInMinPredict_dy_Val]
  Compare To Constant2/1 -> Switch1/2
  Compare To Constant1/1 -> Switch2/2
  Add4/1 -> CutInProb_Calculation/1
  Abs/1 -> Compare To Constant1/1, Switch2/3, Compare To Constant2/1

== system PubIfDecisionTOS_MDL/TOS_20201112/TOS_2012080320/PIL_1029/ObjCutInOut_Prob/ObjectCutIn/CutInProb_Calculate/CutInProb_Calculate_/CutInProb_ScopeConstraint/CutInObjCutoutMov ==
  note: 目标切出
  note: 目标在中心线左侧，向左运动
  note: 目标在中心线右侧，向右运动
  PP_ObjectToCenterLine_vyc : Inport
  ObjectToCenterLine_dy : Inport  Port=2  OutDataTypeStr=single
  Compare To Constant1 : simulink/Logic and Bit Operations/Compare To Constant  relop=>  const=C_TOS_ObjToCenterLine_ConstantVal_Zeros  OutDataTypeStr=boolean
      settings: AttributesFormatString=C_TOS_ObjToCenterLine_ConstantVal_Zeros = 0
  Compare To Constant2 : simulink/Logic and Bit Operations/Compare To Constant  relop=>  const=P_TOS_CutoutObjvyThre_Val  OutDataTypeStr=boolean
      settings: AttributesFormatString=P_TOS_CutoutObjvyThre_Val = 0.1
  Compare To Constant3 : simulink/Logic and Bit Operations/Compare To Constant  relop=<  const=P_TOS_CutoutObjvyThre_NegativeVal  OutDataTypeStr=boolean
      settings: AttributesFormatString=P_TOS_CutoutObjvyThre_NegativeVal = -0.1
  Switch : Switch  Criteria=u2 ~= 0  OutDataTypeStr=single
  CutInObjCutoutMovflg : Outport
  wires:
  Switch/1 -> CutInObjCutoutMovflg/1
  ObjectToCenterLine_dy/1 -> Compare To Constant1/1
  Compare To Constant1/1 -> Switch/2
  PP_ObjectToCenterLine_vyc/1 -> Compare To Constant3/1, Compare To Constant2/1
  Compare To Constant3/1 -> Switch/3
  Compare To Constant2/1 -> Switch/1

== system PubIfDecisionTOS_MDL/TOS_20201112/TOS_2012080320/PIL_1029/ObjCutInOut_Prob/ObjectCutIn/CutInProb_Calculate/CutInProb_Calculate_/CutInProb_ScopeConstraint/CutInObjWidthConstraint ==
  note: 目标进入自车道内；
  note: 目标在中心线左侧
  note: 目标在中心线右侧
  ObjectToCenterLine_dy : Inport  OutDataTypeStr=single
  Object_Width : Inport  Port=2
  Abs2 : Abs
  Add : Sum  Inputs=-+
  Add1 : Sum
  C_HalfWidthVehicle_Con : Constant  Value=C_TOS_HalfWidthVehicle_Con  OutDataTypeStr=single
      settings: AttributesFormatString=C_TOS_HalfWidthVehicle_Con = 0.5
  Compare To Constant2 : simulink/Logic and Bit Operations/Compare To Constant  relop=<=  const=P_TOS_CutinObjectToCenterLine_dy_Val  OutDataTypeStr=boolean
      settings: AttributesFormatString=P_TOS_CutinObjectToCenterLine_dy_Val = 0.1
  Constant3 : Constant  Value=C_TOS_ObjToCenterLine_ConstantVal_Zeros  OutDataTypeStr=single
      settings: AttributesFormatString=C_TOS_ObjToCenterLine_ConstantVal_Zeros = 0
  Max : MinMax  Function=max  Inputs=2  OutDataTypeStr=single
  Max1 : MinMax  Inputs=2  OutDataTypeStr=single
  Product : Product  OutDataTypeStr=single
  Relational Operator : RelationalOperator  Operator=>  OutDataTypeStr=boolean  RndMeth=Nearest
  Switch : Switch  Criteria=u2 > Threshold  OutDataTypeStr=single
  constant1 : Constant  Value=0  OutDataTypeStr=single
  constant2 : Constant  Value=0  OutDataTypeStr=single
  CutInPredictDis_dy_ObjWidthConstraint : Outport
  wires:
  Add1/1 -> Max1/2
  Product/1 -> Add/1, Add1/2
  C_HalfWidthVehicle_Con/1 -> Product/1
  Relational Operator/1 -> Switch/2
  Constant3/1 -> Relational Operator/2
  constant1/1 -> Max/1
  ObjectToCenterLine_dy/1 -> Add/2, Add1/1, Relational Operator/1
  Object_Width/1 -> Product/2
  Max/1 -> Switch/1
  constant2/1 -> Max1/1
  Max1/1 -> Switch/3
  Add/1 -> Max/2
  Switch/1 -> Abs2/1
  Abs2/1 -> Compare To Constant2/1
  Compare To Constant2/1 -> CutInPredictDis_dy_ObjWidthConstraint/1

== system PubIfDecisionTOS_MDL/TOS_20201112/TOS_2012080320/PIL_1029/ObjCutInOut_Prob/ObjectCutIn/CutInProb_Calculate/CutInProb_Calculate_/CutInProb_ScopeConstraint1/ObjectCutinMind1 ==
  PP_ObjectToCenterLine_vyc : Inport  OutDataTypeStr=single
  ObjectToCenterLine_dy : Inport  Port=2  OutDataTypeStr=single
  Object_Width : Inport  Port=3
  Abs1 : Abs
  Compare To Constant2 : simulink/Logic and Bit Operations/Compare To Constant  relop=<=  const=P_TOS_CutinObjvyThre_Val  OutDataTypeStr=boolean
      settings: AttributesFormatString=P_TOS_CutinObjvyThre_Val = 0.06
  CutInObjCutoutMov : Subsystem
  CutInObjWidthConstraint : Subsystem
  Logical Operator1 : Logic  Operator=OR  AllPortsSameDT=off  OutDataTypeStr=boolean
  Logical Operator2 : Logic  Operator=OR  AllPortsSameDT=off  OutDataTypeStr=boolean
  ObjectCutinMindFlg : Outport
  wires:
  Logical Operator2/1 -> ObjectCutinMindFlg/1
  CutInObjWidthConstraint/1(CutInPredictDis_dy_ObjWidthConstraint) -> Logical Operator2/2
  ObjectToCenterLine_dy/1 -> CutInObjWidthConstraint/1(ObjectToCenterLine_dy), CutInObjCutoutMov/2(ObjectToCenterLine_dy)
  PP_ObjectToCenterLine_vyc/1 -> CutInObjCutoutMov/1(PP_ObjectToCenterLine_vyc), Abs1/1
  Compare To Constant2/1 -> Logical Operator1/1
  Abs1/1 -> Compare To Constant2/1
  Object_Width/1 -> CutInObjWidthConstraint/2(Object_Width)
  CutInObjCutoutMov/1(CutInObjCutoutMovflg) -> Logical Operator1/2
  Logical Operator1/1 -> Logical Operator2/1

== system PubIfDecisionTOS_MDL/TOS_20201112/TOS_2012080320/PIL_1029/ObjCutInOut_Prob/ObjectCutIn/CutInProb_Calculate/CutInProb_Calculate_/CutInProb_ScopeConstraint1/ScopeConstraint ==
  note: 调节 cut in 横向范围
  note: 角度范围 [-45° , 45°]
  Object_DX : Inport  OutDataTypeStr=single
  PP_ObjectToCenterLine_dy : Inport  Port=2
  Object_Age : Inport  Port=3
  Abs : Abs
  Abs1 : Abs
  Compare To Constant1 : simulink/Logic and Bit Operations/Compare To Constant  relop=>  const=P_TOS_ObjCutInObject_DY_Val  OutDataTypeStr=boolean
      settings: AttributesFormatString=P_TOS_ObjCutInObject_DY_Val = 2.4
  Compare To Constant2 : simulink/Logic and Bit Operations/Compare To Constant  relop=<  const=C_TOS_Obj_Age_Val  OutDataTypeStr=boolean
      settings: AttributesFormatString=C_TOS_Obj_Age_Val = 1
  Compare To Constant3 : simulink/Logic and Bit Operations/Compare To Constant  relop=>  const=P_TOS_CutInAngleFilt_Val  OutDataTypeStr=boolean
      settings: AttributesFormatString=P_TOS_CutInAngleFilt_Val = 0.25
  Compare To Constant4 : simulink/Logic and Bit Operations/Compare To Constant  relop=>  const=C_TOS_Objdx_Constraint_Val  OutDataTypeStr=boolean
      settings: AttributesFormatString=C_TOS_Objdx_Constraint_Val = 0
  Constant2 : Constant  Value=0  OutDataTypeStr=single
  Divide : Product  Inputs=*/
  Logical Operator1 : Logic  Operator=OR  AllPortsSameDT=off  OutDataTypeStr=boolean
  Saturation : Saturate  UpperLimit=255  LowerLimit=0.01  OutDataTypeStr=single
  Switch1 : Switch  Criteria=u2 > Threshold  OutDataTypeStr=single
  Terminator : Terminator
  ScopeConstraint : Outport
  wires:
  Abs1/1 -> Compare To Constant3/1
  Object_Age/1 -> Compare To Constant2/1
  Compare To Constant1/1 -> Logical Operator1/2
  Divide/1 -> Switch1/1
  PP_ObjectToCenterLine_dy/1 -> Divide/1, Abs/1
  Compare To Constant4/1 -> Switch1/2
  Abs/1 -> Compare To Constant1/1
  Switch1/1 -> Abs1/1
  Compare To Constant2/1 -> Logical Operator1/1
  Constant2/1 -> Switch1/3
  Compare To Constant3/1 -> Terminator/1
  Object_DX/1 -> Compare To Constant4/1, Saturation/1
  Logical Operator1/1 -> ScopeConstraint/1
  Saturation/1 -> Divide/2

== system PubIfDecisionTOS_MDL/TOS_20201112/TOS_2012080320/PIL_1029/ObjCutInOut_Prob/ObjectCutOut/CutOutProb_Calculate/CutOutProb_Calculate/CutOutPredictDis_dy/CutOutPredictTime ==
  note: 非车辆目标，根据 ObjectToCenterLine_dy 定义预测时间
  ObjectToCenterLine_dy_Filt : Inport  OutDataTypeStr=single
  ObjectToCenterLin e_dy : Inport  Port=2  OutDataTypeStr=single
  ObjectType : Inport  Port=3
  PP_ObjectToCenterLine_vyc : Inport  Port=4  OutDataTypeStr=single
  Object_DX : Inport  Port=5
  1-D Lookup Table : Lookup_n-D  NumberOfTableDimensions=1  BreakpointsForDimension1=[0,10,30,100]  Table=[1,1,0.8,0.8]  InternalRulePriority=Speed  RndMeth=Simplest  InputSameDT=on
  CarTruck_ToCenterLine_dy_Predict : Subsystem
  K_CutInMaxPredictTime_Val : Constant  Value=P_TOS_CutOutMaxPredictTime_Val  OutDataTypeStr=single
      settings: AttributesFormatString=P_TOS_CutOutMaxPredictTime_Val = 1.0
  K_CutInMinPredictTime_Val : Constant  Value=P_TOS_CutOutMinPredictTime_Val  OutDataTypeStr=single
      settings: AttributesFormatString=P_TOS_CutOutMinPredictTime_Val = 1
  ObjectToCenterLine_dy_Predict : Subsystem
  Switch : Switch  Criteria=u2 > Threshold  OutDataTypeStr=single
  Switch1 : Switch  Criteria=u2 ~= 0  OutDataTypeStr=single
  CutOutPredictTime : Outport
  wires:
  K_CutInMaxPredictTime_Val/1 -> Switch/1
  K_CutInMinPredictTime_Val/1 -> Switch/3
  Switch/1 -> Switch1/3
  ObjectToCenterLine_dy_Filt/1 -> ObjectToCenterLine_dy_Predict/1(ObjectToCenterLine_dy_Filt)
  ObjectToCenterLin e_dy/1 -> ObjectToCenterLine_dy_Predict/2(ObjectToCenterLine_dy)
  ObjectToCenterLine_dy_Predict/1(CutOutPredictTime) -> Switch/2
  ObjectType/1 -> CarTruck_ToCenterLine_dy_Predict/1(ObjectType)
  PP_ObjectToCenterLine_vyc/1 -> CarTruck_ToCenterLine_dy_Predict/2(PP_ObjectToCenterLine_vyc)
  CarTruck_ToCenterLine_dy_Predict/1(CarTruck_ToCenterLine_dy_Predict) -> Switch1/2
  Switch1/1 -> CutOutPredictTime/1  "CutOutPredictTime"
  1-D Lookup Table/1 -> Switch1/1  "CutOutPredictTime"
  Object_DX/1 -> 1-D Lookup Table/1

== system PubIfDecisionTOS_MDL/TOS_20201112/TOS_2012080320/PIL_1029/ObjCutInOut_Prob/ObjectCutOut/CutOutProb_Calculate/CutOutProb_Calculate/CutOutPredictDis_dy/CutOutPredictTime_Constraint1 ==
  note: 插值计算，根据dx距离 约束预测时间
  note: [  min ,  prt ]
      | [  max , 0   ]
  note: fun:cut in 预测时间约束
      |
      | 根据 dx 约束目标预测时间
  CutOutPredictTime : Inport
  Object_DX : Inport  Port=2
  Add1 : Sum  Inputs=+-  OutDataTypeStr=single
  Add2 : Sum  Inputs=-+  AccumDataTypeStr=single  OutDataTypeStr=single
  Compare To Constant : simulink/Logic and Bit Operations/Compare To Constant  relop=<=  const=P_TOS_CutOutMinPredictDis_Val  OutDataTypeStr=boolean
      settings: AttributesFormatString=P_TOS_CutOutMinPredictDis_Val = 3.93 m
  Compare To Constant1 : simulink/Logic and Bit Operations/Compare To Constant  relop=>=  const=P_TOS_CutOutMaxPredictDis_Val  OutDataTypeStr=boolean
      settings: AttributesFormatString=P_TOS_CutOutMaxPredictDis_Val = 110 m
  Divide : Product  Inputs=*/  OutDataTypeStr=single
  Divide1 : Product  Inputs=**  OutDataTypeStr=single
  Divide2 : Product  Inputs=**  OutDataTypeStr=single
  Divide3 : Product  Inputs=*/  OutDataTypeStr=single
  K_CutInMaxPredictDis_Val : Constant  Value=P_TOS_CutOutMaxPredictDis_Val  OutDataTypeStr=single
      settings: AttributesFormatString=P_TOS_CutOutMaxPredictDis_Val = 110
  K_CutInMinPredictDis_Val : Constant  Value=P_TOS_CutOutMinPredictDis_Val  OutDataTypeStr=single
      settings: AttributesFormatString=P_TOS_CutOutMinPredictDis_Val = 3.93
  Switch1 : Switch  Criteria=u2 > Threshold
  Switch2 : Switch  Criteria=u2 > Threshold
  CutOutPredictTime_Constraint1 : Outport  OutDataTypeStr=single
  wires:
  Add2/1 -> CutOutPredictTime_Constraint1/1
  Divide3/1 -> Add2/1
  [K_CutOutMaxPredictDis_Val] -> Divide2/2
  Divide1/1 -> Add2/2
  Compare To Constant/1 -> Switch1/2
  Switch2/1 -> Switch1/3
  [K_CutOutMinPredictDis_Val] -> Add1/1
  Switch1/1 -> Divide1/2
  K_CutInMinPredictDis_Val/1 -> Switch1/1, [K_CutOutMinPredictDis_Val]
  Divide2/1 -> Divide3/1
  Divide/1 -> Divide1/1
  Object_DX/1 -> Compare To Constant/1, Compare To Constant1/1, Switch2/3
  Compare To Constant1/1 -> Switch2/2
  [K_CutOutMaxPredictDis_Val] -> Add1/2
  CutOutPredictTime/1 -> Divide2/1, Divide/1
  K_CutInMaxPredictDis_Val/1 -> Switch2/1, [K_CutOutMaxPredictDis_Val]
  Add1/1 -> Divide/2, Divide3/2
